simulink model "sinusoidal"  (R2020a)
settings: Solver=VariableStepAuto  StartTime=0.0  StopTime=10.0  RelTol=1e-3
settings Model: Creator=surya  LastModifiedBy=surya

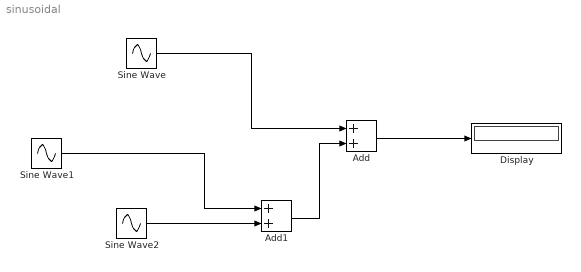
== system sinusoidal ==
  Add : Sum
  Add1 : Sum
  Display : Display
  Sine Wave : Sin  Amplitude=100  SampleTime=0
  Sine Wave1 : Sin  Amplitude=100  SampleTime=0
  Sine Wave2 : Sin  Amplitude=100  SampleTime=0
  wires:
  Sine Wave1/1 -> Add1/1
  Sine Wave2/1 -> Add1/2
  Sine Wave/1 -> Add/1
  Add1/1 -> Add/2
  Add/1 -> Display/1
